simulink model "M3b_mdl"  (R2021b)
settings: Solver=ode45  StartTime=0.0  StopTime=10.0  MaxStep=0.01  RelTol=1e-3
settings Model: Creator=Studenci  LastModifiedBy=Studenci
settings SolverCC: MaxConsecutiveMinStep=50

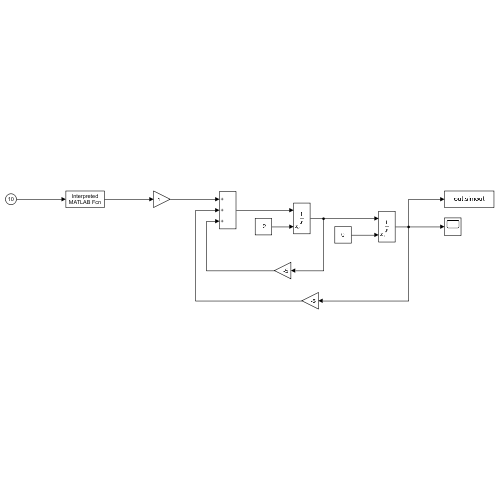
[thumbnail: Simulink's stored preview of the top-level diagram]
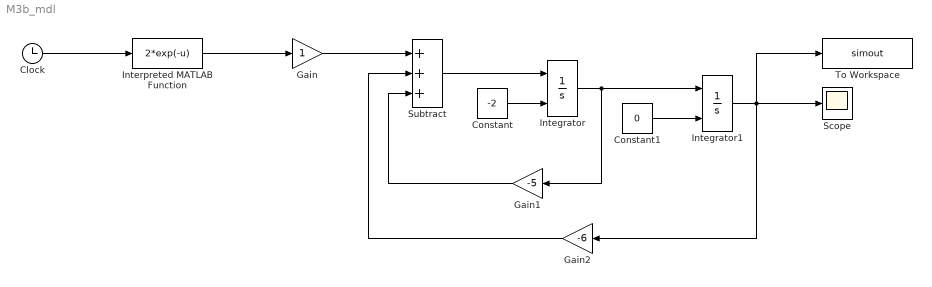
== system M3b_mdl ==
  Clock : Clock
  Constant : Constant  Value=-2
  Constant1 : Constant  Value=0
  Gain : Gain
  Gain1 : Gain  Gain=-5
  Gain2 : Gain  Gain=-6
  Integrator : Integrator  InitialConditionSource=external
  Integrator1 : Integrator  InitialConditionSource=external
  Interpreted MATLAB Function : MATLABFcn  MATLABFcn=2*exp(-u)
  Scope : Scope
  Subtract : Sum  Inputs=+++
  To Workspace : ToWorkspace  VariableName=simout  SaveFormat=Timeseries  SampleTime=-1
  wires:
  Interpreted MATLAB Function/1 -> Gain/1
  Gain/1 -> Subtract/1
  Integrator/1 -> Integrator1/1, Gain1/1
  Constant/1 -> Integrator/2
  Gain1/1 -> Subtract/3
  Subtract/1 -> Integrator/1
  Integrator1/1 -> To Workspace/1, Gain2/1, Scope/1
  Constant1/1 -> Integrator1/2
  Gain2/1 -> Subtract/2
  Clock/1 -> Interpreted MATLAB Function/1
